simulink model "nonlinear_water_tank_model"  (R2017b)
settings: Solver=VariableStepAuto  StartTime=0  StopTime=100  RelTol=1e-3
values from neighbouring files (symbols this model uses):
  hmax = 5    [nonlinear_water_tank.m]
  hp = 0.2    [nonlinear_water_tank.m]
undefined symbols (not defined in the file or in its folder): h0, kmu, kv, mup, rmax
settings Model: Creator=janhauser  LastModifiedBy=janhauser

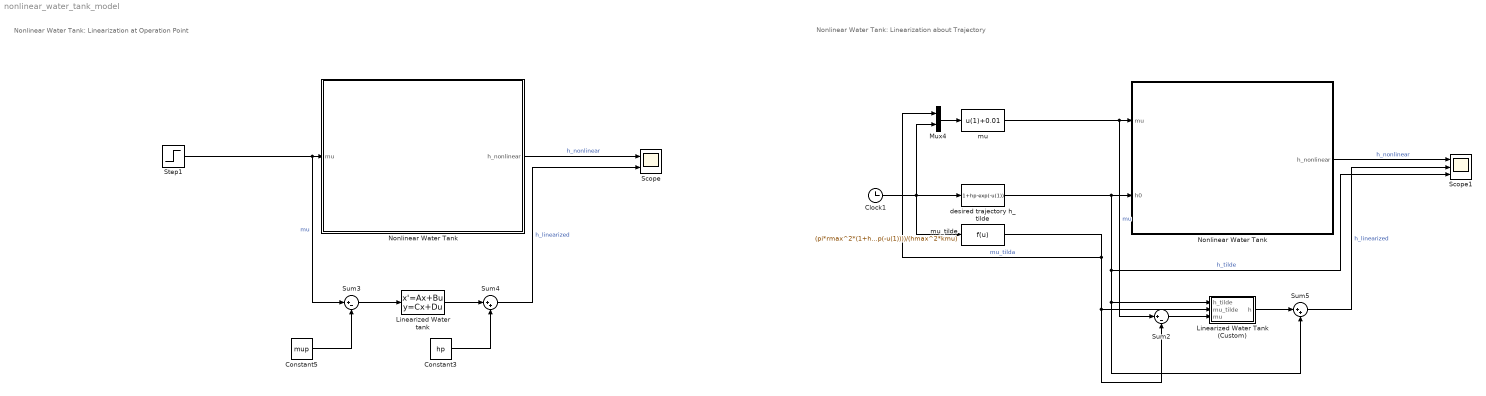
== system nonlinear_water_tank_model ==
  note: Nonlinear Water Tank: Linearization about Trajectory
  note: Nonlinear Water Tank: Linearization at Operation Point
  Clock1 : Clock
  Constant3 : Constant  Value=hp
  Constant5 : Constant  Value=mup
  "Linearized Water Tank (Custom) " : Subsystem
      mask Display: image('/Users/janhauser/Desktop/Screenshot 2019-02-06 at 16.05.31.png');
  Linearized Water tank : StateSpace  A=(- 5/(8*hp^(5/2)*pi) - (20*mup - 5*hp^(1/2))/(2*hp^3*pi))  B=5/(hp^2*pi)  D=0  InitialCondition=0
  Mux4 : Mux  Inputs=2
  Nonlinear Water Tank : Subsystem
      mask Display: image('/Users/janhauser/Desktop/Screenshot 2019-02-05 at 13.33.04.png');
  "Nonlinear Water Tank " : Subsystem
      mask Display: image('/Users/janhauser/Desktop/Screenshot 2019-02-05 at 13.33.04.png');
  Scope : Scope  NumInputPorts=2
  Scope1 : Scope  NumInputPorts=3
  Step1 : Step  Time=0  After=mup+0.01  SampleTime=0
  Sum2 : Sum  Inputs=|+-
  Sum3 : Sum  Inputs=|+-
  Sum4 : Sum  Inputs=|++
  Sum5 : Sum  Inputs=|++
  desired trajectory h_tilde : Fcn  Expr=1+hp-exp(-u(1))
  mu : Fcn  Expr=u(1)+0.01
  mu_tilde : Fcn  Expr=(pi*rmax^2*(1+hp-exp(-u(1)))^2*exp(-u(1))+hmax^2*kv*sqrt(1+hp-exp(-u(1))))/(hmax^2*kmu)
  wires:
  Nonlinear Water Tank/1(h_nonlinear) -> Scope/1  "h_nonlinear"
  Step1/1 -> Sum3/1, Nonlinear Water Tank/1(mu)  "mu"
  Constant3/1 -> Sum4/2
  Constant5/1 -> Sum3/2
  Sum3/1 -> Linearized Water tank/1
  Linearized Water tank/1 -> Sum4/1
  Sum4/1 -> Scope/2  "h_linearized"
  desired trajectory h_tilde/1 -> Sum5/2, "Linearized Water Tank (Custom) "/1(h_tilde), Scope1/3, "Nonlinear Water Tank "/2("h0 ")  "h_tilde"
  "Nonlinear Water Tank "/1(h_nonlinear) -> Scope1/1  "h_nonlinear"
  mu_tilde/1 -> Sum2/2, "Linearized Water Tank (Custom) "/2(mu_tilde), Mux4/1  "mu_tilda"
  Sum5/1 -> Scope1/2  "h_linearized"
  mu/1 -> Sum2/1, "Nonlinear Water Tank "/1(mu)  "mu"
  Sum2/1 -> "Linearized Water Tank (Custom) "/3(mu)
  "Linearized Water Tank (Custom) "/1(h) -> Sum5/1
  Clock1/1 -> mu_tilde/1, Mux4/2, desired trajectory h_tilde/1
  Mux4/1 -> mu/1

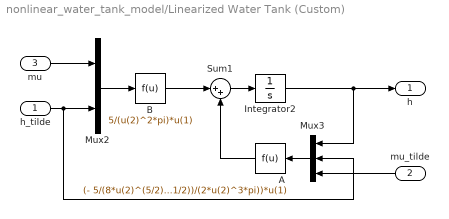
== system nonlinear_water_tank_model/Linearized Water Tank (Custom)  ==
  h_tilde : Inport
  mu_tilde : Inport  Port=2
  mu : Inport  Port=3
  A : Fcn  Expr=(- 5/(8*u(2)^(5/2)*pi) - (20*u(3) - 5*u(2)^(1/2))/(2*u(2)^3*pi))*u(1)
  B : Fcn  Expr=5/(u(2)^2*pi)*u(1)
  Integrator2 : Integrator
  Mux2 : Mux  Inputs=2
  Mux3 : Mux  Inputs=3
  Sum1 : Sum  Inputs=|++
  h : Outport
  wires:
  h_tilde/1 -> Mux2/2, Mux3/2
  mu_tilde/1 -> Mux3/3
  A/1 -> Sum1/2
  Mux3/1 -> A/1
  mu/1 -> Mux2/1
  Mux2/1 -> B/1
  Integrator2/1 -> Mux3/1, h/1
  B/1 -> Sum1/1
  Sum1/1 -> Integrator2/1

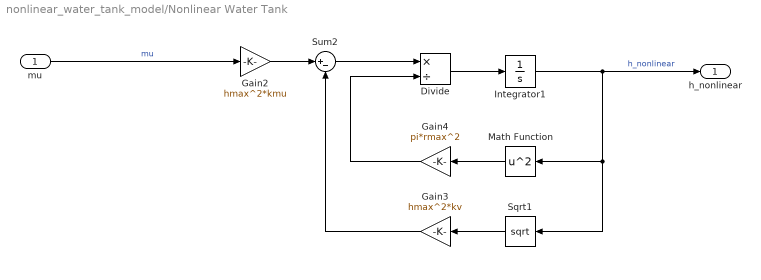
== system nonlinear_water_tank_model/Nonlinear Water Tank ==
  mu : Inport
  Divide : Product  Inputs=*/
  Gain2 : Gain  Gain=hmax^2*kmu
  Gain3 : Gain  Gain=hmax^2*kv
  Gain4 : Gain  Gain=pi*rmax^2
  Integrator1 : Integrator  InitialCondition=hp
  Math Function : Math  Operator=square  SaturateOnIntegerOverflow=on
  Sqrt1 : Sqrt  SaturateOnIntegerOverflow=on
  Sum2 : Sum  Inputs=|+-
  h_nonlinear : Outport
  wires:
  Sum2/1 -> Divide/1
  Gain3/1 -> Sum2/2
  Gain4/1 -> Divide/2
  Math Function/1 -> Gain4/1
  Divide/1 -> Integrator1/1
  Sqrt1/1 -> Gain3/1
  Integrator1/1 -> Math Function/1, Sqrt1/1, h_nonlinear/1  "h_nonlinear"
  Gain2/1 -> Sum2/1
  mu/1 -> Gain2/1  "mu"

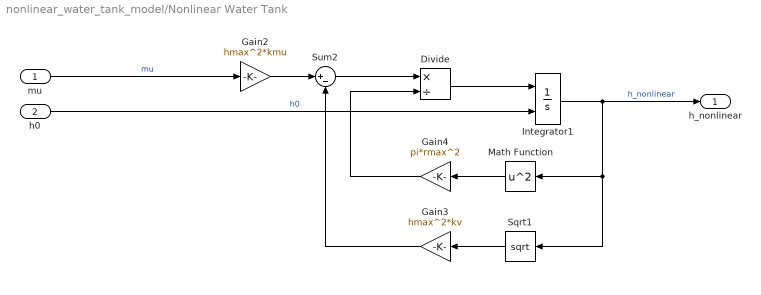
== system nonlinear_water_tank_model/Nonlinear Water Tank  ==
  mu : Inport
  "h0 " : Inport  Port=2
  Divide : Product  Inputs=*/
  Gain2 : Gain  Gain=hmax^2*kmu
  Gain3 : Gain  Gain=hmax^2*kv
  Gain4 : Gain  Gain=pi*rmax^2
  Integrator1 : Integrator  InitialConditionSource=external  InitialCondition=h0
  Math Function : Math  Operator=square  SaturateOnIntegerOverflow=on
  Sqrt1 : Sqrt  SaturateOnIntegerOverflow=on
  Sum2 : Sum  Inputs=|+-
  h_nonlinear : Outport
  wires:
  Sum2/1 -> Divide/1
  Gain3/1 -> Sum2/2
  Gain4/1 -> Divide/2
  Math Function/1 -> Gain4/1
  Divide/1 -> Integrator1/1
  Sqrt1/1 -> Gain3/1
  Integrator1/1 -> Math Function/1, Sqrt1/1, h_nonlinear/1  "h_nonlinear"
  Gain2/1 -> Sum2/1
  mu/1 -> Gain2/1  "mu"
  "h0 "/1 -> Integrator1/2  "h0"
